simulink model "sdof"  (R2015a)
settings: Solver=ode45  StartTime=0.0  StopTime=10.0  FixedStep=0.001  RelTol=1e-3
settings Model: Creator=Aranya Dan  LastModifiedBy=Aranya Dan

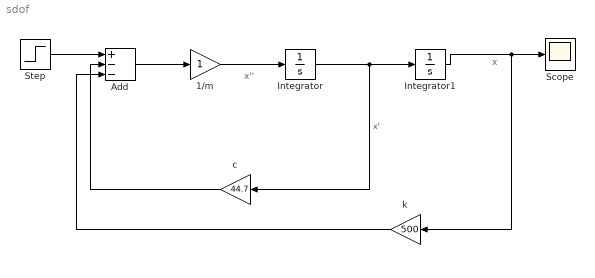
== system sdof ==
  note: x''
  note: x
  1/m : Gain
  Add : Sum  Inputs=+--
  Integrator : Integrator
  Integrator1 : Integrator
  Scope : Scope
  Step : Step  Time=0  SampleTime=0
  c : Gain  Gain=44.7
  k : Gain  Gain=500
  wires:
  Step/1 -> Add/1
  Add/1 -> 1/m/1
  Integrator/1 -> c/1, Integrator1/1  "x'"
  Integrator1/1 -> k/1, Scope/1
  1/m/1 -> Integrator/1
  c/1 -> Add/2
  k/1 -> Add/3
